simulink model "pattern3x3_training_2023clock"  (R2024a)
settings: Solver=FixedStepAuto  StartTime=0.0  StopTime=2  FixedStep=0.000005  RelTol=1e-3
model workspace (MAT data in the model file):
  part1_v1 = 1
values from neighbouring files (symbols this model uses):
  full_pattern = load('Pattern4_250.CSV')    [model_setup4.m]
  max_weight2 = 255    [model_setup4.m]
  min_weight2 = 150    [model_setup4.m]
  Th_minus_count2 = 10    [model_setup4.m]    (also in model_setup_test.m = 5)
  Th_plus_count2 = 20    [model_setup4.m]    (also in model_setup_test.m)
libraries: simulink x1
(part 5 of 9)

== system pattern3x3_training_2023clock/Neuron4/Clock4 ==
  clock : Inport
  "Reset " : Inport  Port=2
  Memory2 : Memory
  NOT1 : Logic  Operator=NOT  IconShape=distinctive  AllPortsSameDT=off  OutDataTypeStr=boolean
  Product1 : Product
  Scope4 : Scope  NumInputPorts=4
  Triggered Subsystem1 : Subsystem  TreatAsAtomicUnit=on
  T : Outport  VectorParamsAs1DForOutWhenUnconnected=off
  wires:
  Memory2/1 -> Triggered Subsystem1/1(In1)
  Product1/1 -> Scope4/4, T/1, Memory2/1
  "Reset "/1 -> Scope4/2, NOT1/1
  Triggered Subsystem1/1(Out1) -> Scope4/3, Product1/1
  NOT1/1 -> Product1/2
  clock/1 -> Scope4/1, Triggered Subsystem1/Trigger

== system pattern3x3_training_2023clock/Neuron4/Subsystem2 ==
  note: 기존 membrane potential + input potential
  Input potential : Inport
  before_Potential : Inport  Port=2
  Trigger : TriggerPort  VariantControl=(inherit)  PortDimensions=1
  Sum : Sum  Inputs=|++
  membrane_state : Outport
  wires:
  Input potential/1 -> Sum/1
  Sum/1 -> membrane_state/1
  before_Potential/1 -> Sum/2

== system pattern3x3_training_2023clock/Neuron4/Subsystem3 ==
  spike : Inport  OutDataTypeStr=double
  initial_threshold : Inport  Port=2
  neuron_num : Inport  Port=3
  clock : Inport  Port=4
  Add1 : Sum
  Constant2 : Constant  Value=0
  Delay : Delay  DelayLength=1  SampleTime=0.00001
  Delay1 : Delay  DelayLength=1  SampleTime=0.00001
  From Workspace3 : FromWorkspace  VariableName=Th_plus
  From Workspace4 : FromWorkspace  VariableName=Th_minus
  From Workspace5 : FromWorkspace  VariableName=Th_mean_count
  From Workspace6 : FromWorkspace  VariableName=min_th
  From Workspace7 : FromWorkspace  VariableName=max_th
  MATLAB Function : MATLAB Function  TreatAsAtomicUnit=on
  MATLAB Function2 : MATLAB Function  TreatAsAtomicUnit=on
  Memory2 : Memory
  NOT : Logic  Operator=NOT  IconShape=distinctive  AllPortsSameDT=off  OutDataTypeStr=boolean
  Product : Product
  Product1 : Product
  Scope1 : Scope  NumInputPorts=3
  Scope2 : Scope  NumInputPorts=3
  Scope3 : Scope  NumInputPorts=3
  Scope4 : Scope  NumInputPorts=4
  Sum : Sum  Inputs=++|
  Sum1 : Sum  Inputs=|++
  Switch3 : Switch  Criteria=u2 > Threshold  SaturateOnIntegerOverflow=off  InputSameDT=off
  Switch4 : Switch  Threshold=Th_plus_count2  SaturateOnIntegerOverflow=off  InputSameDT=off
  Switch5 : Switch  Threshold=Th_minus_count2  SaturateOnIntegerOverflow=off  InputSameDT=off
  clock_0.02 : Subsystem
  spike_generator2 : Subsystem
  Threshold : Outport
  wires:
  MATLAB Function2/1(y) -> Scope3/1, Sum/2
  Sum/1 -> MATLAB Function/1(u)  "Threshold"
  From Workspace7/1 -> MATLAB Function/3(max)
  Delay1/1 -> Scope3/3, MATLAB Function2/3(before_threshold)
  neuron_num/1 -> MATLAB Function2/2(neuron_num)
  MATLAB Function/1(y) -> Delay1/1, Scope3/2, Threshold/1
  initial_threshold/1 -> MATLAB Function2/1(init_th)
  From Workspace6/1 -> MATLAB Function/2(min)
  clock_0.02/1(clock) -> Switch3/2, Scope4/1, Product1/1, NOT/1
  Product1/1 -> Scope2/2, Scope4/2, spike_generator2/1(del_th)
  spike/1 -> Scope2/1, Sum1/1
  Delay/1 -> Sum1/2
  Product/1 -> Delay/1, Scope2/3
  Switch4/1 -> Add1/1, Scope1/1
  Switch5/1 -> Scope1/3, Add1/2
  Sum1/1 -> Product1/2, Product/2
  Constant2/1 -> Switch5/1, Switch4/3
  From Workspace4/1 -> Switch5/3
  Switch3/1 -> Scope4/4, Switch5/2, Switch4/2
  From Workspace3/1 -> Switch4/1
  NOT/1 -> Product/1
  spike_generator2/1(del_th_spike) -> Switch3/1, Scope4/3
  From Workspace5/1 -> Switch3/3
  Memory2/1 -> Scope1/2, Sum/1
  Add1/1 -> Memory2/1
  clock/1 -> clock_0.02/1(In1)

== system pattern3x3_training_2023clock/Neuron4/spike_generator1 ==
  1 : Inport
  AND : Logic  IconShape=distinctive  AllPortsSameDT=off  OutDataTypeStr=boolean
  Cast To Double : DataTypeConversion  OutDataTypeStr=double  SaturateOnIntegerOverflow=off  RndMeth=Floor
  Delay1 : Delay
  NOT : Logic  Operator=NOT  IconShape=distinctive  AllPortsSameDT=off  OutDataTypeStr=boolean
  Scope3 : Scope  NumInputPorts=5
  spike : Outport
  wires:
  NOT/1 -> Scope3/2, Delay1/1
  Delay1/1 -> Scope3/3, AND/2
  AND/1 -> Scope3/4, Cast To Double/1
  1/1 -> AND/1, Scope3/1, NOT/1
  Cast To Double/1 -> Scope3/5, spike/1

== system pattern3x3_training_2023clock/Neuron5/Clock4 ==
  clock : Inport
  "Reset " : Inport  Port=2
  Memory2 : Memory
  NOT1 : Logic  Operator=NOT  IconShape=distinctive  AllPortsSameDT=off  OutDataTypeStr=boolean
  Product1 : Product
  Scope4 : Scope  NumInputPorts=4
  Triggered Subsystem1 : Subsystem  TreatAsAtomicUnit=on
  T : Outport  VectorParamsAs1DForOutWhenUnconnected=off
  wires:
  Memory2/1 -> Triggered Subsystem1/1(In1)
  Product1/1 -> Scope4/4, T/1, Memory2/1
  "Reset "/1 -> Scope4/2, NOT1/1
  Triggered Subsystem1/1(Out1) -> Scope4/3, Product1/1
  NOT1/1 -> Product1/2
  clock/1 -> Scope4/1, Triggered Subsystem1/Trigger

== system pattern3x3_training_2023clock/Neuron5/Subsystem2 ==
  note: 기존 membrane potential + input potential
  Input potential : Inport
  before_Potential : Inport  Port=2
  Trigger : TriggerPort  VariantControl=(inherit)  PortDimensions=1
  Sum : Sum  Inputs=|++
  membrane_state : Outport
  wires:
  Input potential/1 -> Sum/1
  Sum/1 -> membrane_state/1
  before_Potential/1 -> Sum/2

== system pattern3x3_training_2023clock/Neuron5/Subsystem3 ==
  spike : Inport  OutDataTypeStr=double
  initial_threshold : Inport  Port=2
  neuron_num : Inport  Port=3
  clock : Inport  Port=4
  Add1 : Sum
  Constant2 : Constant  Value=0
  Delay : Delay  DelayLength=1  SampleTime=0.00001
  Delay1 : Delay  DelayLength=1  SampleTime=0.00001
  From Workspace3 : FromWorkspace  VariableName=Th_plus
  From Workspace4 : FromWorkspace  VariableName=Th_minus
  From Workspace5 : FromWorkspace  VariableName=Th_mean_count
  From Workspace6 : FromWorkspace  VariableName=min_th
  From Workspace7 : FromWorkspace  VariableName=max_th
  MATLAB Function : MATLAB Function  TreatAsAtomicUnit=on
  MATLAB Function2 : MATLAB Function  TreatAsAtomicUnit=on
  Memory2 : Memory
  NOT : Logic  Operator=NOT  IconShape=distinctive  AllPortsSameDT=off  OutDataTypeStr=boolean
  Product : Product
  Product1 : Product
  Scope1 : Scope  NumInputPorts=3
  Scope2 : Scope  NumInputPorts=3
  Scope3 : Scope  NumInputPorts=3
  Scope4 : Scope  NumInputPorts=4
  Sum : Sum  Inputs=++|
  Sum1 : Sum  Inputs=|++
  Switch3 : Switch  Criteria=u2 > Threshold  SaturateOnIntegerOverflow=off  InputSameDT=off
  Switch4 : Switch  Threshold=Th_plus_count2  SaturateOnIntegerOverflow=off  InputSameDT=off
  Switch5 : Switch  Threshold=Th_minus_count2  SaturateOnIntegerOverflow=off  InputSameDT=off
  clock_0.02 : Subsystem
  spike_generator2 : Subsystem
  Threshold : Outport
  wires:
  MATLAB Function2/1(y) -> Scope3/1, Sum/2
  Sum/1 -> MATLAB Function/1(u)  "Threshold"
  From Workspace7/1 -> MATLAB Function/3(max)
  Delay1/1 -> Scope3/3, MATLAB Function2/3(before_threshold)
  neuron_num/1 -> MATLAB Function2/2(neuron_num)
  MATLAB Function/1(y) -> Delay1/1, Scope3/2, Threshold/1
  initial_threshold/1 -> MATLAB Function2/1(init_th)
  From Workspace6/1 -> MATLAB Function/2(min)
  clock_0.02/1(clock) -> Switch3/2, Scope4/1, Product1/1, NOT/1
  Product1/1 -> Scope2/2, Scope4/2, spike_generator2/1(del_th)
  spike/1 -> Scope2/1, Sum1/1
  Delay/1 -> Sum1/2
  Product/1 -> Delay/1, Scope2/3
  Switch4/1 -> Add1/1, Scope1/1
  Switch5/1 -> Scope1/3, Add1/2
  Sum1/1 -> Product1/2, Product/2
  Constant2/1 -> Switch5/1, Switch4/3
  From Workspace4/1 -> Switch5/3
  Switch3/1 -> Scope4/4, Switch5/2, Switch4/2
  From Workspace3/1 -> Switch4/1
  NOT/1 -> Product/1
  spike_generator2/1(del_th_spike) -> Switch3/1, Scope4/3
  From Workspace5/1 -> Switch3/3
  Memory2/1 -> Scope1/2, Sum/1
  Add1/1 -> Memory2/1
  clock/1 -> clock_0.02/1(In1)

== system pattern3x3_training_2023clock/Neuron5/spike_generator1 ==
  1 : Inport
  AND : Logic  IconShape=distinctive  AllPortsSameDT=off  OutDataTypeStr=boolean
  Cast To Double : DataTypeConversion  OutDataTypeStr=double  SaturateOnIntegerOverflow=off  RndMeth=Floor
  Delay1 : Delay
  NOT : Logic  Operator=NOT  IconShape=distinctive  AllPortsSameDT=off  OutDataTypeStr=boolean
  Scope3 : Scope  NumInputPorts=5
  spike : Outport
  wires:
  NOT/1 -> Scope3/2, Delay1/1
  Delay1/1 -> Scope3/3, AND/2
  AND/1 -> Scope3/4, Cast To Double/1
  1/1 -> AND/1, Scope3/1, NOT/1
  Cast To Double/1 -> Scope3/5, spike/1

== system pattern3x3_training_2023clock/Neuron6/Clock4 ==
  clock : Inport
  "Reset " : Inport  Port=2
  Memory2 : Memory
  NOT1 : Logic  Operator=NOT  IconShape=distinctive  AllPortsSameDT=off  OutDataTypeStr=boolean
  Product1 : Product
  Scope4 : Scope  NumInputPorts=4
  Triggered Subsystem1 : Subsystem  TreatAsAtomicUnit=on
  T : Outport  VectorParamsAs1DForOutWhenUnconnected=off
  wires:
  Memory2/1 -> Triggered Subsystem1/1(In1)
  Product1/1 -> Scope4/4, T/1, Memory2/1
  "Reset "/1 -> Scope4/2, NOT1/1
  Triggered Subsystem1/1(Out1) -> Scope4/3, Product1/1
  NOT1/1 -> Product1/2
  clock/1 -> Scope4/1, Triggered Subsystem1/Trigger

== system pattern3x3_training_2023clock/Neuron6/Subsystem2 ==
  note: 기존 membrane potential + input potential
  Input potential : Inport
  before_Potential : Inport  Port=2
  Trigger : TriggerPort  VariantControl=(inherit)  PortDimensions=1
  Sum : Sum  Inputs=|++
  membrane_state : Outport
  wires:
  Input potential/1 -> Sum/1
  Sum/1 -> membrane_state/1
  before_Potential/1 -> Sum/2

== system pattern3x3_training_2023clock/Neuron6/Subsystem3 ==
  spike : Inport  OutDataTypeStr=double
  initial_threshold : Inport  Port=2
  neuron_num : Inport  Port=3
  clock : Inport  Port=4
  Add1 : Sum
  Constant2 : Constant  Value=0
  Delay : Delay  DelayLength=1  SampleTime=0.00001
  Delay1 : Delay  DelayLength=1  SampleTime=0.00001
  From Workspace3 : FromWorkspace  VariableName=Th_plus
  From Workspace4 : FromWorkspace  VariableName=Th_minus
  From Workspace5 : FromWorkspace  VariableName=Th_mean_count
  From Workspace6 : FromWorkspace  VariableName=min_th
  From Workspace7 : FromWorkspace  VariableName=max_th
  MATLAB Function : MATLAB Function  TreatAsAtomicUnit=on
  MATLAB Function2 : MATLAB Function  TreatAsAtomicUnit=on
  Memory2 : Memory
  NOT : Logic  Operator=NOT  IconShape=distinctive  AllPortsSameDT=off  OutDataTypeStr=boolean
  Product : Product
  Product1 : Product
  Scope1 : Scope  NumInputPorts=3
  Scope2 : Scope  NumInputPorts=3
  Scope3 : Scope  NumInputPorts=3
  Scope4 : Scope  NumInputPorts=4
  Sum : Sum  Inputs=++|
  Sum1 : Sum  Inputs=|++
  Switch3 : Switch  Criteria=u2 > Threshold  SaturateOnIntegerOverflow=off  InputSameDT=off
  Switch4 : Switch  Threshold=Th_plus_count2  SaturateOnIntegerOverflow=off  InputSameDT=off
  Switch5 : Switch  Threshold=Th_minus_count2  SaturateOnIntegerOverflow=off  InputSameDT=off
  clock_0.02 : Subsystem
  spike_generator2 : Subsystem
  Threshold : Outport
  wires:
  MATLAB Function2/1(y) -> Scope3/1, Sum/2
  Sum/1 -> MATLAB Function/1(u)  "Threshold"
  From Workspace7/1 -> MATLAB Function/3(max)
  Delay1/1 -> Scope3/3, MATLAB Function2/3(before_threshold)
  neuron_num/1 -> MATLAB Function2/2(neuron_num)
  MATLAB Function/1(y) -> Delay1/1, Scope3/2, Threshold/1
  initial_threshold/1 -> MATLAB Function2/1(init_th)
  From Workspace6/1 -> MATLAB Function/2(min)
  clock_0.02/1(clock) -> Switch3/2, Scope4/1, Product1/1, NOT/1
  Product1/1 -> Scope2/2, Scope4/2, spike_generator2/1(del_th)
  spike/1 -> Scope2/1, Sum1/1
  Delay/1 -> Sum1/2
  Product/1 -> Delay/1, Scope2/3
  Switch4/1 -> Add1/1, Scope1/1
  Switch5/1 -> Scope1/3, Add1/2
  Sum1/1 -> Product1/2, Product/2
  Constant2/1 -> Switch5/1, Switch4/3
  From Workspace4/1 -> Switch5/3
  Switch3/1 -> Scope4/4, Switch5/2, Switch4/2
  From Workspace3/1 -> Switch4/1
  NOT/1 -> Product/1
  spike_generator2/1(del_th_spike) -> Switch3/1, Scope4/3
  From Workspace5/1 -> Switch3/3
  Memory2/1 -> Scope1/2, Sum/1
  Add1/1 -> Memory2/1
  clock/1 -> clock_0.02/1(In1)

== system pattern3x3_training_2023clock/Neuron6/spike_generator1 ==
  1 : Inport
  AND : Logic  IconShape=distinctive  AllPortsSameDT=off  OutDataTypeStr=boolean
  Cast To Double : DataTypeConversion  OutDataTypeStr=double  SaturateOnIntegerOverflow=off  RndMeth=Floor
  Delay1 : Delay
  NOT : Logic  Operator=NOT  IconShape=distinctive  AllPortsSameDT=off  OutDataTypeStr=boolean
  Scope3 : Scope  NumInputPorts=5
  spike : Outport
  wires:
  NOT/1 -> Scope3/2, Delay1/1
  Delay1/1 -> Scope3/3, AND/2
  AND/1 -> Scope3/4, Cast To Double/1
  1/1 -> AND/1, Scope3/1, NOT/1
  Cast To Double/1 -> Scope3/5, spike/1

== system pattern3x3_training_2023clock/Neuron7/Clock4 ==
  clock : Inport
  "Reset " : Inport  Port=2
  Memory2 : Memory
  NOT1 : Logic  Operator=NOT  IconShape=distinctive  AllPortsSameDT=off  OutDataTypeStr=boolean
  Product1 : Product
  Scope4 : Scope  NumInputPorts=4
  Triggered Subsystem1 : Subsystem  TreatAsAtomicUnit=on
  T : Outport  VectorParamsAs1DForOutWhenUnconnected=off
  wires:
  Memory2/1 -> Triggered Subsystem1/1(In1)
  Product1/1 -> Scope4/4, T/1, Memory2/1
  "Reset "/1 -> Scope4/2, NOT1/1
  Triggered Subsystem1/1(Out1) -> Scope4/3, Product1/1
  NOT1/1 -> Product1/2
  clock/1 -> Scope4/1, Triggered Subsystem1/Trigger

== system pattern3x3_training_2023clock/Neuron7/Subsystem2 ==
  note: 기존 membrane potential + input potential
  Input potential : Inport
  before_Potential : Inport  Port=2
  Trigger : TriggerPort  VariantControl=(inherit)  PortDimensions=1
  Sum : Sum  Inputs=|++
  membrane_state : Outport
  wires:
  Input potential/1 -> Sum/1
  Sum/1 -> membrane_state/1
  before_Potential/1 -> Sum/2

== system pattern3x3_training_2023clock/Neuron7/Subsystem3 ==
  spike : Inport  OutDataTypeStr=double
  initial_threshold : Inport  Port=2
  neuron_num : Inport  Port=3
  clock : Inport  Port=4
  Add1 : Sum
  Constant2 : Constant  Value=0
  Delay : Delay  DelayLength=1  SampleTime=0.00001
  Delay1 : Delay  DelayLength=1  SampleTime=0.00001
  From Workspace3 : FromWorkspace  VariableName=Th_plus
  From Workspace4 : FromWorkspace  VariableName=Th_minus
  From Workspace5 : FromWorkspace  VariableName=Th_mean_count
  From Workspace6 : FromWorkspace  VariableName=min_th
  From Workspace7 : FromWorkspace  VariableName=max_th
  MATLAB Function : MATLAB Function  TreatAsAtomicUnit=on
  MATLAB Function2 : MATLAB Function  TreatAsAtomicUnit=on
  Memory2 : Memory
  NOT : Logic  Operator=NOT  IconShape=distinctive  AllPortsSameDT=off  OutDataTypeStr=boolean
  Product : Product
  Product1 : Product
  Scope1 : Scope  NumInputPorts=3
  Scope2 : Scope  NumInputPorts=3
  Scope3 : Scope  NumInputPorts=3
  Scope4 : Scope  NumInputPorts=4
  Sum : Sum  Inputs=++|
  Sum1 : Sum  Inputs=|++
  Switch3 : Switch  Criteria=u2 > Threshold  SaturateOnIntegerOverflow=off  InputSameDT=off
  Switch4 : Switch  Threshold=Th_plus_count2  SaturateOnIntegerOverflow=off  InputSameDT=off
  Switch5 : Switch  Threshold=Th_minus_count2  SaturateOnIntegerOverflow=off  InputSameDT=off
  clock_0.02 : Subsystem
  spike_generator2 : Subsystem
  Threshold : Outport
  wires:
  MATLAB Function2/1(y) -> Scope3/1, Sum/2
  Sum/1 -> MATLAB Function/1(u)  "Threshold"
  From Workspace7/1 -> MATLAB Function/3(max)
  Delay1/1 -> Scope3/3, MATLAB Function2/3(before_threshold)
  neuron_num/1 -> MATLAB Function2/2(neuron_num)
  MATLAB Function/1(y) -> Delay1/1, Scope3/2, Threshold/1
  initial_threshold/1 -> MATLAB Function2/1(init_th)
  From Workspace6/1 -> MATLAB Function/2(min)
  clock_0.02/1(clock) -> Switch3/2, Scope4/1, Product1/1, NOT/1
  Product1/1 -> Scope2/2, Scope4/2, spike_generator2/1(del_th)
  spike/1 -> Scope2/1, Sum1/1
  Delay/1 -> Sum1/2
  Product/1 -> Delay/1, Scope2/3
  Switch4/1 -> Add1/1, Scope1/1
  Switch5/1 -> Scope1/3, Add1/2
  Sum1/1 -> Product1/2, Product/2
  Constant2/1 -> Switch5/1, Switch4/3
  From Workspace4/1 -> Switch5/3
  Switch3/1 -> Scope4/4, Switch5/2, Switch4/2
  From Workspace3/1 -> Switch4/1
  NOT/1 -> Product/1
  spike_generator2/1(del_th_spike) -> Switch3/1, Scope4/3
  From Workspace5/1 -> Switch3/3
  Memory2/1 -> Scope1/2, Sum/1
  Add1/1 -> Memory2/1
  clock/1 -> clock_0.02/1(In1)

== system pattern3x3_training_2023clock/Neuron7/spike_generator1 ==
  1 : Inport
  AND : Logic  IconShape=distinctive  AllPortsSameDT=off  OutDataTypeStr=boolean
  Cast To Double : DataTypeConversion  OutDataTypeStr=double  SaturateOnIntegerOverflow=off  RndMeth=Floor
  Delay1 : Delay
  NOT : Logic  Operator=NOT  IconShape=distinctive  AllPortsSameDT=off  OutDataTypeStr=boolean
  Scope3 : Scope  NumInputPorts=5
  spike : Outport
  wires:
  NOT/1 -> Scope3/2, Delay1/1
  Delay1/1 -> Scope3/3, AND/2
  AND/1 -> Scope3/4, Cast To Double/1
  1/1 -> AND/1, Scope3/1, NOT/1
  Cast To Double/1 -> Scope3/5, spike/1

== system pattern3x3_training_2023clock/Neuron8/Clock4 ==
  clock : Inport
  "Reset " : Inport  Port=2
  Memory2 : Memory
  NOT1 : Logic  Operator=NOT  IconShape=distinctive  AllPortsSameDT=off  OutDataTypeStr=boolean
  Product1 : Product
  Scope4 : Scope  NumInputPorts=4
  Triggered Subsystem1 : Subsystem  TreatAsAtomicUnit=on
  T : Outport  VectorParamsAs1DForOutWhenUnconnected=off
  wires:
  Memory2/1 -> Triggered Subsystem1/1(In1)
  Product1/1 -> Scope4/4, T/1, Memory2/1
  "Reset "/1 -> Scope4/2, NOT1/1
  Triggered Subsystem1/1(Out1) -> Scope4/3, Product1/1
  NOT1/1 -> Product1/2
  clock/1 -> Scope4/1, Triggered Subsystem1/Trigger

== system pattern3x3_training_2023clock/Neuron8/Subsystem2 ==
  note: 기존 membrane potential + input potential
  Input potential : Inport
  before_Potential : Inport  Port=2
  Trigger : TriggerPort  VariantControl=(inherit)  PortDimensions=1
  Sum : Sum  Inputs=|++
  membrane_state : Outport
  wires:
  Input potential/1 -> Sum/1
  Sum/1 -> membrane_state/1
  before_Potential/1 -> Sum/2

== system pattern3x3_training_2023clock/Neuron8/Subsystem3 ==
  spike : Inport  OutDataTypeStr=double
  initial_threshold : Inport  Port=2
  neuron_num : Inport  Port=3
  clock : Inport  Port=4
  Add1 : Sum
  Constant2 : Constant  Value=0
  Delay : Delay  DelayLength=1  SampleTime=0.00001
  Delay1 : Delay  DelayLength=1  SampleTime=0.00001
  From Workspace3 : FromWorkspace  VariableName=Th_plus
  From Workspace4 : FromWorkspace  VariableName=Th_minus
  From Workspace5 : FromWorkspace  VariableName=Th_mean_count
  From Workspace6 : FromWorkspace  VariableName=min_th
  From Workspace7 : FromWorkspace  VariableName=max_th
  MATLAB Function : MATLAB Function  TreatAsAtomicUnit=on
  MATLAB Function2 : MATLAB Function  TreatAsAtomicUnit=on
  Memory2 : Memory
  NOT : Logic  Operator=NOT  IconShape=distinctive  AllPortsSameDT=off  OutDataTypeStr=boolean
  Product : Product
  Product1 : Product
  Scope1 : Scope  NumInputPorts=3
  Scope2 : Scope  NumInputPorts=3
  Scope3 : Scope  NumInputPorts=3
  Scope4 : Scope  NumInputPorts=4
  Sum : Sum  Inputs=++|
  Sum1 : Sum  Inputs=|++
  Switch3 : Switch  Criteria=u2 > Threshold  SaturateOnIntegerOverflow=off  InputSameDT=off
  Switch4 : Switch  Threshold=Th_plus_count2  SaturateOnIntegerOverflow=off  InputSameDT=off
  Switch5 : Switch  Threshold=Th_minus_count2  SaturateOnIntegerOverflow=off  InputSameDT=off
  clock_0.02 : Subsystem
  spike_generator2 : Subsystem
  Threshold : Outport
  wires:
  MATLAB Function2/1(y) -> Scope3/1, Sum/2
  Sum/1 -> MATLAB Function/1(u)  "Threshold"
  From Workspace7/1 -> MATLAB Function/3(max)
  Delay1/1 -> Scope3/3, MATLAB Function2/3(before_threshold)
  neuron_num/1 -> MATLAB Function2/2(neuron_num)
  MATLAB Function/1(y) -> Delay1/1, Scope3/2, Threshold/1
  initial_threshold/1 -> MATLAB Function2/1(init_th)
  From Workspace6/1 -> MATLAB Function/2(min)
  clock_0.02/1(clock) -> Switch3/2, Scope4/1, Product1/1, NOT/1
  Product1/1 -> Scope2/2, Scope4/2, spike_generator2/1(del_th)
  spike/1 -> Scope2/1, Sum1/1
  Delay/1 -> Sum1/2
  Product/1 -> Delay/1, Scope2/3
  Switch4/1 -> Add1/1, Scope1/1
  Switch5/1 -> Scope1/3, Add1/2
  Sum1/1 -> Product1/2, Product/2
  Constant2/1 -> Switch5/1, Switch4/3
  From Workspace4/1 -> Switch5/3
  Switch3/1 -> Scope4/4, Switch5/2, Switch4/2
  From Workspace3/1 -> Switch4/1
  NOT/1 -> Product/1
  spike_generator2/1(del_th_spike) -> Switch3/1, Scope4/3
  From Workspace5/1 -> Switch3/3
  Memory2/1 -> Scope1/2, Sum/1
  Add1/1 -> Memory2/1
  clock/1 -> clock_0.02/1(In1)

== system pattern3x3_training_2023clock/Neuron8/spike_generator1 ==
  1 : Inport
  AND : Logic  IconShape=distinctive  AllPortsSameDT=off  OutDataTypeStr=boolean
  Cast To Double : DataTypeConversion  OutDataTypeStr=double  SaturateOnIntegerOverflow=off  RndMeth=Floor
  Delay1 : Delay
  NOT : Logic  Operator=NOT  IconShape=distinctive  AllPortsSameDT=off  OutDataTypeStr=boolean
  Scope3 : Scope  NumInputPorts=5
  spike : Outport
  wires:
  NOT/1 -> Scope3/2, Delay1/1
  Delay1/1 -> Scope3/3, AND/2
  AND/1 -> Scope3/4, Cast To Double/1
  1/1 -> AND/1, Scope3/1, NOT/1
  Cast To Double/1 -> Scope3/5, spike/1

== system pattern3x3_training_2023clock/Neuron9/Clock4 ==
  clock : Inport
  "Reset " : Inport  Port=2
  Memory2 : Memory
  NOT1 : Logic  Operator=NOT  IconShape=distinctive  AllPortsSameDT=off  OutDataTypeStr=boolean
  Product1 : Product
  Scope4 : Scope  NumInputPorts=4
  Triggered Subsystem1 : Subsystem  TreatAsAtomicUnit=on
  T : Outport  VectorParamsAs1DForOutWhenUnconnected=off
  wires:
  Memory2/1 -> Triggered Subsystem1/1(In1)
  Product1/1 -> Scope4/4, T/1, Memory2/1
  "Reset "/1 -> Scope4/2, NOT1/1
  Triggered Subsystem1/1(Out1) -> Scope4/3, Product1/1
  NOT1/1 -> Product1/2
  clock/1 -> Scope4/1, Triggered Subsystem1/Trigger

== system pattern3x3_training_2023clock/Neuron9/Subsystem2 ==
  note: 기존 membrane potential + input potential
  Input potential : Inport
  before_Potential : Inport  Port=2
  Trigger : TriggerPort  VariantControl=(inherit)  PortDimensions=1
  Sum : Sum  Inputs=|++
  membrane_state : Outport
  wires:
  Input potential/1 -> Sum/1
  Sum/1 -> membrane_state/1
  before_Potential/1 -> Sum/2

== system pattern3x3_training_2023clock/Neuron9/Subsystem3 ==
  spike : Inport  OutDataTypeStr=double
  initial_threshold : Inport  Port=2
  neuron_num : Inport  Port=3
  clock : Inport  Port=4
  Add1 : Sum
  Constant2 : Constant  Value=0
  Delay : Delay  DelayLength=1  SampleTime=0.00001
  Delay1 : Delay  DelayLength=1  SampleTime=0.00001
  From Workspace3 : FromWorkspace  VariableName=Th_plus
  From Workspace4 : FromWorkspace  VariableName=Th_minus
  From Workspace5 : FromWorkspace  VariableName=Th_mean_count
  From Workspace6 : FromWorkspace  VariableName=min_th
  From Workspace7 : FromWorkspace  VariableName=max_th
  MATLAB Function : MATLAB Function  TreatAsAtomicUnit=on
  MATLAB Function2 : MATLAB Function  TreatAsAtomicUnit=on
  Memory2 : Memory
  NOT : Logic  Operator=NOT  IconShape=distinctive  AllPortsSameDT=off  OutDataTypeStr=boolean
  Product : Product
  Product1 : Product
  Scope1 : Scope  NumInputPorts=3
  Scope2 : Scope  NumInputPorts=3
  Scope3 : Scope  NumInputPorts=3
  Scope4 : Scope  NumInputPorts=4
  Sum : Sum  Inputs=++|
  Sum1 : Sum  Inputs=|++
  Switch3 : Switch  Criteria=u2 > Threshold  SaturateOnIntegerOverflow=off  InputSameDT=off
  Switch4 : Switch  Threshold=Th_plus_count2  SaturateOnIntegerOverflow=off  InputSameDT=off
  Switch5 : Switch  Threshold=Th_minus_count2  SaturateOnIntegerOverflow=off  InputSameDT=off
  clock_0.02 : Subsystem
  spike_generator2 : Subsystem
  Threshold : Outport
  wires:
  MATLAB Function2/1(y) -> Scope3/1, Sum/2
  Sum/1 -> MATLAB Function/1(u)  "Threshold"
  From Workspace7/1 -> MATLAB Function/3(max)
  Delay1/1 -> Scope3/3, MATLAB Function2/3(before_threshold)
  neuron_num/1 -> MATLAB Function2/2(neuron_num)
  MATLAB Function/1(y) -> Delay1/1, Scope3/2, Threshold/1
  initial_threshold/1 -> MATLAB Function2/1(init_th)
  From Workspace6/1 -> MATLAB Function/2(min)
  clock_0.02/1(clock) -> Switch3/2, Scope4/1, Product1/1, NOT/1
  Product1/1 -> Scope2/2, Scope4/2, spike_generator2/1(del_th)
  spike/1 -> Scope2/1, Sum1/1
  Delay/1 -> Sum1/2
  Product/1 -> Delay/1, Scope2/3
  Switch4/1 -> Add1/1, Scope1/1
  Switch5/1 -> Scope1/3, Add1/2
  Sum1/1 -> Product1/2, Product/2
  Constant2/1 -> Switch5/1, Switch4/3
  From Workspace4/1 -> Switch5/3
  Switch3/1 -> Scope4/4, Switch5/2, Switch4/2
  From Workspace3/1 -> Switch4/1
  NOT/1 -> Product/1
  spike_generator2/1(del_th_spike) -> Switch3/1, Scope4/3
  From Workspace5/1 -> Switch3/3
  Memory2/1 -> Scope1/2, Sum/1
  Add1/1 -> Memory2/1
  clock/1 -> clock_0.02/1(In1)

== system pattern3x3_training_2023clock/Neuron9/spike_generator1 ==
  1 : Inport
  AND : Logic  IconShape=distinctive  AllPortsSameDT=off  OutDataTypeStr=boolean
  Cast To Double : DataTypeConversion  OutDataTypeStr=double  SaturateOnIntegerOverflow=off  RndMeth=Floor
  Delay1 : Delay
  NOT : Logic  Operator=NOT  IconShape=distinctive  AllPortsSameDT=off  OutDataTypeStr=boolean
  Scope3 : Scope  NumInputPorts=5
  spike : Outport
  wires:
  NOT/1 -> Scope3/2, Delay1/1
  Delay1/1 -> Scope3/3, AND/2
  AND/1 -> Scope3/4, Cast To Double/1
  1/1 -> AND/1, Scope3/1, NOT/1
  Cast To Double/1 -> Scope3/5, spike/1

== system pattern3x3_training_2023clock/Post_Neuron1/Clock1 ==
  clock : Inport
  "Reset " : Inport  Port=2
  Memory2 : Memory
  NOT1 : Logic  Operator=NOT  IconShape=distinctive  AllPortsSameDT=off  OutDataTypeStr=boolean
  Product1 : Product
  Triggered Subsystem1 : Subsystem  TreatAsAtomicUnit=on
  T : Outport  VectorParamsAs1DForOutWhenUnconnected=off
  wires:
  Memory2/1 -> Triggered Subsystem1/1(In1)
  Product1/1 -> T/1, Memory2/1
  "Reset "/1 -> NOT1/1
  Triggered Subsystem1/1(Out1) -> Product1/1
  NOT1/1 -> Product1/2
  clock/1 -> Triggered Subsystem1/Trigger

== system pattern3x3_training_2023clock/Post_Neuron1/Clock2 ==
  clock : Inport
  "Reset " : Inport  Port=2
  Memory2 : Memory
  NOT1 : Logic  Operator=NOT  IconShape=distinctive  AllPortsSameDT=off  OutDataTypeStr=boolean
  Product1 : Product
  Triggered Subsystem1 : Subsystem  TreatAsAtomicUnit=on
  T : Outport  VectorParamsAs1DForOutWhenUnconnected=off
  wires:
  Memory2/1 -> Triggered Subsystem1/1(In1)
  Product1/1 -> T/1, Memory2/1
  "Reset "/1 -> NOT1/1
  Triggered Subsystem1/1(Out1) -> Product1/1
  NOT1/1 -> Product1/2
  clock/1 -> Triggered Subsystem1/Trigger

== system pattern3x3_training_2023clock/Post_Neuron1/Subsystem1 ==
  In1 : Inport
  In2 : Inport  Port=2
  Trigger : TriggerPort  VariantControl=(inherit)  PortDimensions=1
  Sum : Sum  Inputs=|++
  membrane_state : Outport
  wires:
  In1/1 -> Sum/1
  Sum/1 -> membrane_state/1
  In2/1 -> Sum/2

== system pattern3x3_training_2023clock/Post_Neuron1/Subsystem3 ==
  spike : Inport  OutDataTypeStr=double
  initial_threshold : Inport  Port=2
  neuron_num : Inport  Port=3
  clock : Inport  Port=4
  Add1 : Sum
  Constant2 : Constant  Value=0
  Delay : Delay  DelayLength=1  SampleTime=0.00001
  Delay1 : Delay  DelayLength=1  SampleTime=0.00001
  From Workspace3 : FromWorkspace  VariableName=Th_plus
  From Workspace4 : FromWorkspace  VariableName=Th_minus
  From Workspace5 : FromWorkspace  VariableName=Th_mean_count
  From Workspace6 : FromWorkspace  VariableName=min_th
  From Workspace7 : FromWorkspace  VariableName=max_th
  MATLAB Function : MATLAB Function  TreatAsAtomicUnit=on
  MATLAB Function2 : MATLAB Function  TreatAsAtomicUnit=on
  Memory2 : Memory
  NOT : Logic  Operator=NOT  IconShape=distinctive  AllPortsSameDT=off  OutDataTypeStr=boolean
  Product : Product
  Product1 : Product
  Scope1 : Scope  NumInputPorts=3
  Scope2 : Scope  NumInputPorts=3
  Scope3 : Scope  NumInputPorts=3
  Scope4 : Scope  NumInputPorts=4
  Sum : Sum  Inputs=++|
  Sum1 : Sum  Inputs=|++
  Switch3 : Switch  Criteria=u2 > Threshold  SaturateOnIntegerOverflow=off  InputSameDT=off
  Switch4 : Switch  Threshold=Th_plus_count2  SaturateOnIntegerOverflow=off  InputSameDT=off
  Switch5 : Switch  Threshold=Th_minus_count2  SaturateOnIntegerOverflow=off  InputSameDT=off
  clock_0.02 : Subsystem
  spike_generator2 : Subsystem
  Threshold : Outport
  wires:
  MATLAB Function2/1(y) -> Scope3/1, Sum/2
  Sum/1 -> MATLAB Function/1(u)  "Threshold"
  From Workspace7/1 -> MATLAB Function/3(max)
  Delay1/1 -> Scope3/3, MATLAB Function2/3(before_threshold)
  neuron_num/1 -> MATLAB Function2/2(neuron_num)
  MATLAB Function/1(y) -> Delay1/1, Scope3/2, Threshold/1
  initial_threshold/1 -> MATLAB Function2/1(init_th)
  From Workspace6/1 -> MATLAB Function/2(min)
  clock_0.02/1(clock) -> Switch3/2, Scope4/1, Product1/1, NOT/1
  Product1/1 -> Scope2/2, Scope4/2, spike_generator2/1(del_th)
  spike/1 -> Scope2/1, Sum1/1
  Delay/1 -> Sum1/2
  Product/1 -> Delay/1, Scope2/3
  Switch4/1 -> Add1/1, Scope1/1
  Switch5/1 -> Scope1/3, Add1/2
  Sum1/1 -> Product1/2, Product/2
  Constant2/1 -> Switch5/1, Switch4/3
  From Workspace4/1 -> Switch5/3
  Switch3/1 -> Scope4/4, Switch5/2, Switch4/2
  From Workspace3/1 -> Switch4/1
  NOT/1 -> Product/1
  spike_generator2/1(del_th_spike) -> Switch3/1, Scope4/3
  From Workspace5/1 -> Switch3/3
  Memory2/1 -> Scope1/2, Sum/1
  Add1/1 -> Memory2/1
  clock/1 -> clock_0.02/1(In1)

== system pattern3x3_training_2023clock/Post_Neuron1/memory ==
  In1 : Inport
  Memory2 : Memory
  Memory4 : Memory
  OR : Logic  Operator=OR  IconShape=distinctive  AllPortsSameDT=off  OutDataTypeStr=boolean
  Out1 : Outport
  wires:
  Memory4/1 -> Memory2/1, OR/1
  Memory2/1 -> OR/2
  OR/1 -> Out1/1
  In1/1 -> Memory4/1

== system pattern3x3_training_2023clock/Post_Neuron1/spike_generator1 ==
  1 : Inport
  AND : Logic  IconShape=distinctive  AllPortsSameDT=off  OutDataTypeStr=boolean
  Cast To Double : DataTypeConversion  OutDataTypeStr=double  SaturateOnIntegerOverflow=off  RndMeth=Floor
  Delay1 : Delay
  NOT : Logic  Operator=NOT  IconShape=distinctive  AllPortsSameDT=off  OutDataTypeStr=boolean
  Scope3 : Scope  NumInputPorts=5
  spike : Outport
  wires:
  NOT/1 -> Scope3/2, Delay1/1
  Delay1/1 -> Scope3/3, AND/2
  AND/1 -> Scope3/4, Cast To Double/1
  1/1 -> AND/1, Scope3/1, NOT/1
  Cast To Double/1 -> Scope3/5, spike/1

== system pattern3x3_training_2023clock/Post_Neuron2/Clock1 ==
  clock : Inport
  "Reset " : Inport  Port=2
  Memory2 : Memory
  NOT1 : Logic  Operator=NOT  IconShape=distinctive  AllPortsSameDT=off  OutDataTypeStr=boolean
  Product1 : Product
  Triggered Subsystem1 : Subsystem  TreatAsAtomicUnit=on
  T : Outport  VectorParamsAs1DForOutWhenUnconnected=off
  wires:
  Memory2/1 -> Triggered Subsystem1/1(In1)
  Product1/1 -> T/1, Memory2/1
  "Reset "/1 -> NOT1/1
  Triggered Subsystem1/1(Out1) -> Product1/1
  NOT1/1 -> Product1/2
  clock/1 -> Triggered Subsystem1/Trigger

== system pattern3x3_training_2023clock/Post_Neuron2/Clock2 ==
  clock : Inport
  "Reset " : Inport  Port=2
  Memory2 : Memory
  NOT1 : Logic  Operator=NOT  IconShape=distinctive  AllPortsSameDT=off  OutDataTypeStr=boolean
  Product1 : Product
  Triggered Subsystem1 : Subsystem  TreatAsAtomicUnit=on
  T : Outport  VectorParamsAs1DForOutWhenUnconnected=off
  wires:
  Memory2/1 -> Triggered Subsystem1/1(In1)
  Product1/1 -> T/1, Memory2/1
  "Reset "/1 -> NOT1/1
  Triggered Subsystem1/1(Out1) -> Product1/1
  NOT1/1 -> Product1/2
  clock/1 -> Triggered Subsystem1/Trigger

== system pattern3x3_training_2023clock/Post_Neuron2/Subsystem1 ==
  In1 : Inport
  In2 : Inport  Port=2
  Trigger : TriggerPort  VariantControl=(inherit)  PortDimensions=1
  Sum : Sum  Inputs=|++
  membrane_state : Outport
  wires:
  In1/1 -> Sum/1
  Sum/1 -> membrane_state/1
  In2/1 -> Sum/2

== system pattern3x3_training_2023clock/Post_Neuron2/Subsystem3 ==
  spike : Inport  OutDataTypeStr=double
  initial_threshold : Inport  Port=2
  neuron_num : Inport  Port=3
  clock : Inport  Port=4
  Add1 : Sum
  Constant2 : Constant  Value=0
  Delay : Delay  DelayLength=1  SampleTime=0.00001
  Delay1 : Delay  DelayLength=1  SampleTime=0.00001
  From Workspace3 : FromWorkspace  VariableName=Th_plus
  From Workspace4 : FromWorkspace  VariableName=Th_minus
  From Workspace5 : FromWorkspace  VariableName=Th_mean_count
  From Workspace6 : FromWorkspace  VariableName=min_th
  From Workspace7 : FromWorkspace  VariableName=max_th
  MATLAB Function : MATLAB Function  TreatAsAtomicUnit=on
  MATLAB Function2 : MATLAB Function  TreatAsAtomicUnit=on
  Memory2 : Memory
  NOT : Logic  Operator=NOT  IconShape=distinctive  AllPortsSameDT=off  OutDataTypeStr=boolean
  Product : Product
  Product1 : Product
  Scope1 : Scope  NumInputPorts=3
  Scope2 : Scope  NumInputPorts=3
  Scope3 : Scope  NumInputPorts=3
  Scope4 : Scope  NumInputPorts=4
  Sum : Sum  Inputs=++|
  Sum1 : Sum  Inputs=|++
  Switch3 : Switch  Criteria=u2 > Threshold  SaturateOnIntegerOverflow=off  InputSameDT=off
  Switch4 : Switch  Threshold=Th_plus_count2  SaturateOnIntegerOverflow=off  InputSameDT=off
  Switch5 : Switch  Threshold=Th_minus_count2  SaturateOnIntegerOverflow=off  InputSameDT=off
  clock_0.02 : Subsystem
  spike_generator2 : Subsystem
  Threshold : Outport
  wires:
  MATLAB Function2/1(y) -> Scope3/1, Sum/2
  Sum/1 -> MATLAB Function/1(u)  "Threshold"
  From Workspace7/1 -> MATLAB Function/3(max)
  Delay1/1 -> Scope3/3, MATLAB Function2/3(before_threshold)
  neuron_num/1 -> MATLAB Function2/2(neuron_num)
  MATLAB Function/1(y) -> Delay1/1, Scope3/2, Threshold/1
  initial_threshold/1 -> MATLAB Function2/1(init_th)
  From Workspace6/1 -> MATLAB Function/2(min)
  clock_0.02/1(clock) -> Switch3/2, Scope4/1, Product1/1, NOT/1
  Product1/1 -> Scope2/2, Scope4/2, spike_generator2/1(del_th)
  spike/1 -> Scope2/1, Sum1/1
  Delay/1 -> Sum1/2
  Product/1 -> Delay/1, Scope2/3
  Switch4/1 -> Add1/1, Scope1/1
  Switch5/1 -> Scope1/3, Add1/2
  Sum1/1 -> Product1/2, Product/2
  Constant2/1 -> Switch5/1, Switch4/3
  From Workspace4/1 -> Switch5/3
  Switch3/1 -> Scope4/4, Switch5/2, Switch4/2
  From Workspace3/1 -> Switch4/1
  NOT/1 -> Product/1
  spike_generator2/1(del_th_spike) -> Switch3/1, Scope4/3
  From Workspace5/1 -> Switch3/3
  Memory2/1 -> Scope1/2, Sum/1
  Add1/1 -> Memory2/1
  clock/1 -> clock_0.02/1(In1)

== system pattern3x3_training_2023clock/Post_Neuron2/memory ==
  In1 : Inport
  Memory2 : Memory
  Memory4 : Memory
  OR : Logic  Operator=OR  IconShape=distinctive  AllPortsSameDT=off  OutDataTypeStr=boolean
  Out1 : Outport
  wires:
  Memory4/1 -> Memory2/1, OR/1
  Memory2/1 -> OR/2
  OR/1 -> Out1/1
  In1/1 -> Memory4/1

== system pattern3x3_training_2023clock/Post_Neuron2/spike_generator1 ==
  1 : Inport
  AND : Logic  IconShape=distinctive  AllPortsSameDT=off  OutDataTypeStr=boolean
  Cast To Double : DataTypeConversion  OutDataTypeStr=double  SaturateOnIntegerOverflow=off  RndMeth=Floor
  Delay1 : Delay
  NOT : Logic  Operator=NOT  IconShape=distinctive  AllPortsSameDT=off  OutDataTypeStr=boolean
  Scope3 : Scope  NumInputPorts=5
  spike : Outport
  wires:
  NOT/1 -> Scope3/2, Delay1/1
  Delay1/1 -> Scope3/3, AND/2
  AND/1 -> Scope3/4, Cast To Double/1
  1/1 -> AND/1, Scope3/1, NOT/1
  Cast To Double/1 -> Scope3/5, spike/1

== system pattern3x3_training_2023clock/Post_Neuron3/Clock1 ==
  clock : Inport
  "Reset " : Inport  Port=2
  Memory2 : Memory
  NOT1 : Logic  Operator=NOT  IconShape=distinctive  AllPortsSameDT=off  OutDataTypeStr=boolean
  Product1 : Product
  Triggered Subsystem1 : Subsystem  TreatAsAtomicUnit=on
  T : Outport  VectorParamsAs1DForOutWhenUnconnected=off
  wires:
  Memory2/1 -> Triggered Subsystem1/1(In1)
  Product1/1 -> T/1, Memory2/1
  "Reset "/1 -> NOT1/1
  Triggered Subsystem1/1(Out1) -> Product1/1
  NOT1/1 -> Product1/2
  clock/1 -> Triggered Subsystem1/Trigger

== system pattern3x3_training_2023clock/Post_Neuron3/Clock2 ==
  clock : Inport
  "Reset " : Inport  Port=2
  Memory2 : Memory
  NOT1 : Logic  Operator=NOT  IconShape=distinctive  AllPortsSameDT=off  OutDataTypeStr=boolean
  Product1 : Product
  Triggered Subsystem1 : Subsystem  TreatAsAtomicUnit=on
  T : Outport  VectorParamsAs1DForOutWhenUnconnected=off
  wires:
  Memory2/1 -> Triggered Subsystem1/1(In1)
  Product1/1 -> T/1, Memory2/1
  "Reset "/1 -> NOT1/1
  Triggered Subsystem1/1(Out1) -> Product1/1
  NOT1/1 -> Product1/2
  clock/1 -> Triggered Subsystem1/Trigger

== system pattern3x3_training_2023clock/Post_Neuron3/Subsystem1 ==
  In1 : Inport
  In2 : Inport  Port=2
  Trigger : TriggerPort  VariantControl=(inherit)  PortDimensions=1
  Sum : Sum  Inputs=|++
  membrane_state : Outport
  wires:
  In1/1 -> Sum/1
  Sum/1 -> membrane_state/1
  In2/1 -> Sum/2

== system pattern3x3_training_2023clock/Post_Neuron3/Subsystem3 ==
  spike : Inport  OutDataTypeStr=double
  initial_threshold : Inport  Port=2
  neuron_num : Inport  Port=3
  clock : Inport  Port=4
  Add1 : Sum
  Constant2 : Constant  Value=0
  Delay : Delay  DelayLength=1  SampleTime=0.00001
  Delay1 : Delay  DelayLength=1  SampleTime=0.00001
  From Workspace3 : FromWorkspace  VariableName=Th_plus
  From Workspace4 : FromWorkspace  VariableName=Th_minus
  From Workspace5 : FromWorkspace  VariableName=Th_mean_count
  From Workspace6 : FromWorkspace  VariableName=min_th
  From Workspace7 : FromWorkspace  VariableName=max_th
  MATLAB Function : MATLAB Function  TreatAsAtomicUnit=on
  MATLAB Function2 : MATLAB Function  TreatAsAtomicUnit=on
  Memory2 : Memory
  NOT : Logic  Operator=NOT  IconShape=distinctive  AllPortsSameDT=off  OutDataTypeStr=boolean
  Product : Product
  Product1 : Product
  Scope1 : Scope  NumInputPorts=3
  Scope2 : Scope  NumInputPorts=3
  Scope3 : Scope  NumInputPorts=3
  Scope4 : Scope  NumInputPorts=4
  Sum : Sum  Inputs=++|
  Sum1 : Sum  Inputs=|++
  Switch3 : Switch  Criteria=u2 > Threshold  SaturateOnIntegerOverflow=off  InputSameDT=off
  Switch4 : Switch  Threshold=Th_plus_count2  SaturateOnIntegerOverflow=off  InputSameDT=off
  Switch5 : Switch  Threshold=Th_minus_count2  SaturateOnIntegerOverflow=off  InputSameDT=off
  clock_0.02 : Subsystem
  spike_generator2 : Subsystem
  Threshold : Outport
  wires:
  MATLAB Function2/1(y) -> Scope3/1, Sum/2
  Sum/1 -> MATLAB Function/1(u)  "Threshold"
  From Workspace7/1 -> MATLAB Function/3(max)
  Delay1/1 -> Scope3/3, MATLAB Function2/3(before_threshold)
  neuron_num/1 -> MATLAB Function2/2(neuron_num)
  MATLAB Function/1(y) -> Delay1/1, Scope3/2, Threshold/1
  initial_threshold/1 -> MATLAB Function2/1(init_th)
  From Workspace6/1 -> MATLAB Function/2(min)
  clock_0.02/1(clock) -> Switch3/2, Scope4/1, Product1/1, NOT/1
  Product1/1 -> Scope2/2, Scope4/2, spike_generator2/1(del_th)
  spike/1 -> Scope2/1, Sum1/1
  Delay/1 -> Sum1/2
  Product/1 -> Delay/1, Scope2/3
  Switch4/1 -> Add1/1, Scope1/1
  Switch5/1 -> Scope1/3, Add1/2
  Sum1/1 -> Product1/2, Product/2
  Constant2/1 -> Switch5/1, Switch4/3
  From Workspace4/1 -> Switch5/3
  Switch3/1 -> Scope4/4, Switch5/2, Switch4/2
  From Workspace3/1 -> Switch4/1
  NOT/1 -> Product/1
  spike_generator2/1(del_th_spike) -> Switch3/1, Scope4/3
  From Workspace5/1 -> Switch3/3
  Memory2/1 -> Scope1/2, Sum/1
  Add1/1 -> Memory2/1
  clock/1 -> clock_0.02/1(In1)

== system pattern3x3_training_2023clock/Post_Neuron3/memory ==
  In1 : Inport
  Memory2 : Memory
  Memory4 : Memory
  OR : Logic  Operator=OR  IconShape=distinctive  AllPortsSameDT=off  OutDataTypeStr=boolean
  Out1 : Outport
  wires:
  Memory4/1 -> Memory2/1, OR/1
  Memory2/1 -> OR/2
  OR/1 -> Out1/1
  In1/1 -> Memory4/1

== system pattern3x3_training_2023clock/Post_Neuron3/spike_generator1 ==
  1 : Inport
  AND : Logic  IconShape=distinctive  AllPortsSameDT=off  OutDataTypeStr=boolean
  Cast To Double : DataTypeConversion  OutDataTypeStr=double  SaturateOnIntegerOverflow=off  RndMeth=Floor
  Delay1 : Delay
  NOT : Logic  Operator=NOT  IconShape=distinctive  AllPortsSameDT=off  OutDataTypeStr=boolean
  Scope3 : Scope  NumInputPorts=5
  spike : Outport
  wires:
  NOT/1 -> Scope3/2, Delay1/1
  Delay1/1 -> Scope3/3, AND/2
  AND/1 -> Scope3/4, Cast To Double/1
  1/1 -> AND/1, Scope3/1, NOT/1
  Cast To Double/1 -> Scope3/5, spike/1

== system pattern3x3_training_2023clock/Post_Neuron4/Clock1 ==
  clock : Inport
  "Reset " : Inport  Port=2
  Memory2 : Memory
  NOT1 : Logic  Operator=NOT  IconShape=distinctive  AllPortsSameDT=off  OutDataTypeStr=boolean
  Product1 : Product
  Triggered Subsystem1 : Subsystem  TreatAsAtomicUnit=on
  T : Outport  VectorParamsAs1DForOutWhenUnconnected=off
  wires:
  Memory2/1 -> Triggered Subsystem1/1(In1)
  Product1/1 -> T/1, Memory2/1
  "Reset "/1 -> NOT1/1
  Triggered Subsystem1/1(Out1) -> Product1/1
  NOT1/1 -> Product1/2
  clock/1 -> Triggered Subsystem1/Trigger

== system pattern3x3_training_2023clock/Post_Neuron4/Clock2 ==
  clock : Inport
  "Reset " : Inport  Port=2
  Memory2 : Memory
  NOT1 : Logic  Operator=NOT  IconShape=distinctive  AllPortsSameDT=off  OutDataTypeStr=boolean
  Product1 : Product
  Triggered Subsystem1 : Subsystem  TreatAsAtomicUnit=on
  T : Outport  VectorParamsAs1DForOutWhenUnconnected=off
  wires:
  Memory2/1 -> Triggered Subsystem1/1(In1)
  Product1/1 -> T/1, Memory2/1
  "Reset "/1 -> NOT1/1
  Triggered Subsystem1/1(Out1) -> Product1/1
  NOT1/1 -> Product1/2
  clock/1 -> Triggered Subsystem1/Trigger

== system pattern3x3_training_2023clock/Post_Neuron4/Subsystem1 ==
  In1 : Inport
  In2 : Inport  Port=2
  Trigger : TriggerPort  VariantControl=(inherit)  PortDimensions=1
  Sum : Sum  Inputs=|++
  membrane_state : Outport
  wires:
  In1/1 -> Sum/1
  Sum/1 -> membrane_state/1
  In2/1 -> Sum/2

== system pattern3x3_training_2023clock/Post_Neuron4/Subsystem3 ==
  spike : Inport  OutDataTypeStr=double
  initial_threshold : Inport  Port=2
  neuron_num : Inport  Port=3
  clock : Inport  Port=4
  Add1 : Sum
  Constant2 : Constant  Value=0
  Delay : Delay  DelayLength=1  SampleTime=0.00001
  Delay1 : Delay  DelayLength=1  SampleTime=0.00001
  From Workspace3 : FromWorkspace  VariableName=Th_plus
  From Workspace4 : FromWorkspace  VariableName=Th_minus
  From Workspace5 : FromWorkspace  VariableName=Th_mean_count
  From Workspace6 : FromWorkspace  VariableName=min_th
  From Workspace7 : FromWorkspace  VariableName=max_th
  MATLAB Function : MATLAB Function  TreatAsAtomicUnit=on
  MATLAB Function2 : MATLAB Function  TreatAsAtomicUnit=on
  Memory2 : Memory
  NOT : Logic  Operator=NOT  IconShape=distinctive  AllPortsSameDT=off  OutDataTypeStr=boolean
  Product : Product
  Product1 : Product
  Scope1 : Scope  NumInputPorts=3
  Scope2 : Scope  NumInputPorts=3
  Scope3 : Scope  NumInputPorts=3
  Scope4 : Scope  NumInputPorts=4
  Sum : Sum  Inputs=++|
  Sum1 : Sum  Inputs=|++
  Switch3 : Switch  Criteria=u2 > Threshold  SaturateOnIntegerOverflow=off  InputSameDT=off
  Switch4 : Switch  Threshold=Th_plus_count2  SaturateOnIntegerOverflow=off  InputSameDT=off
  Switch5 : Switch  Threshold=Th_minus_count2  SaturateOnIntegerOverflow=off  InputSameDT=off
  clock_0.02 : Subsystem
  spike_generator2 : Subsystem
  Threshold : Outport
  wires:
  MATLAB Function2/1(y) -> Scope3/1, Sum/2
  Sum/1 -> MATLAB Function/1(u)  "Threshold"
  From Workspace7/1 -> MATLAB Function/3(max)
  Delay1/1 -> Scope3/3, MATLAB Function2/3(before_threshold)
  neuron_num/1 -> MATLAB Function2/2(neuron_num)
  MATLAB Function/1(y) -> Delay1/1, Scope3/2, Threshold/1
  initial_threshold/1 -> MATLAB Function2/1(init_th)
  From Workspace6/1 -> MATLAB Function/2(min)
  clock_0.02/1(clock) -> Switch3/2, Scope4/1, Product1/1, NOT/1
  Product1/1 -> Scope2/2, Scope4/2, spike_generator2/1(del_th)
  spike/1 -> Scope2/1, Sum1/1
  Delay/1 -> Sum1/2
  Product/1 -> Delay/1, Scope2/3
  Switch4/1 -> Add1/1, Scope1/1
  Switch5/1 -> Scope1/3, Add1/2
  Sum1/1 -> Product1/2, Product/2
  Constant2/1 -> Switch5/1, Switch4/3
  From Workspace4/1 -> Switch5/3
  Switch3/1 -> Scope4/4, Switch5/2, Switch4/2
  From Workspace3/1 -> Switch4/1
  NOT/1 -> Product/1
  spike_generator2/1(del_th_spike) -> Switch3/1, Scope4/3
  From Workspace5/1 -> Switch3/3
  Memory2/1 -> Scope1/2, Sum/1
  Add1/1 -> Memory2/1
  clock/1 -> clock_0.02/1(In1)

== system pattern3x3_training_2023clock/Post_Neuron4/memory ==
  In1 : Inport
  Memory2 : Memory
  Memory4 : Memory
  OR : Logic  Operator=OR  IconShape=distinctive  AllPortsSameDT=off  OutDataTypeStr=boolean
  Out1 : Outport
  wires:
  Memory4/1 -> Memory2/1, OR/1
  Memory2/1 -> OR/2
  OR/1 -> Out1/1
  In1/1 -> Memory4/1

== system pattern3x3_training_2023clock/Post_Neuron4/spike_generator1 ==
  1 : Inport
  AND : Logic  IconShape=distinctive  AllPortsSameDT=off  OutDataTypeStr=boolean
  Cast To Double : DataTypeConversion  OutDataTypeStr=double  SaturateOnIntegerOverflow=off  RndMeth=Floor
  Delay1 : Delay
  NOT : Logic  Operator=NOT  IconShape=distinctive  AllPortsSameDT=off  OutDataTypeStr=boolean
  Scope3 : Scope  NumInputPorts=5
  spike : Outport
  wires:
  NOT/1 -> Scope3/2, Delay1/1
  Delay1/1 -> Scope3/3, AND/2
  AND/1 -> Scope3/4, Cast To Double/1
  1/1 -> AND/1, Scope3/1, NOT/1
  Cast To Double/1 -> Scope3/5, spike/1

== system pattern3x3_training_2023clock/Synapse1/Clock1 ==
  clock : Inport
  "Reset " : Inport  Port=2
  Memory2 : Memory
  NOT1 : Logic  Operator=NOT  IconShape=distinctive  AllPortsSameDT=off  OutDataTypeStr=boolean
  Product1 : Product
  Triggered Subsystem1 : Subsystem  TreatAsAtomicUnit=on
  T : Outport  VectorParamsAs1DForOutWhenUnconnected=off
  wires:
  Memory2/1 -> Triggered Subsystem1/1(In1)
  Product1/1 -> T/1, Memory2/1
  "Reset "/1 -> NOT1/1
  Triggered Subsystem1/1(Out1) -> Product1/1
  NOT1/1 -> Product1/2
  clock/1 -> Triggered Subsystem1/Trigger

== system pattern3x3_training_2023clock/Synapse1/Clock2 ==
  clock : Inport
  "Reset " : Inport  Port=2
  Memory2 : Memory
  NOT1 : Logic  Operator=NOT  IconShape=distinctive  AllPortsSameDT=off  OutDataTypeStr=boolean
  Product1 : Product
  Triggered Subsystem1 : Subsystem  TreatAsAtomicUnit=on
  T : Outport  VectorParamsAs1DForOutWhenUnconnected=off
  wires:
  Memory2/1 -> Triggered Subsystem1/1(In1)
  Product1/1 -> T/1, Memory2/1
  "Reset "/1 -> NOT1/1
  Triggered Subsystem1/1(Out1) -> Product1/1
  NOT1/1 -> Product1/2
  clock/1 -> Triggered Subsystem1/Trigger

== system pattern3x3_training_2023clock/Synapse1/Clock3 ==
  clock : Inport
  "Reset " : Inport  Port=2
  Memory2 : Memory
  NOT1 : Logic  Operator=NOT  IconShape=distinctive  AllPortsSameDT=off  OutDataTypeStr=boolean
  Product1 : Product
  Triggered Subsystem1 : Subsystem  TreatAsAtomicUnit=on
  T : Outport  VectorParamsAs1DForOutWhenUnconnected=off
  wires:
  Memory2/1 -> Triggered Subsystem1/1(In1)
  Product1/1 -> T/1, Memory2/1
  "Reset "/1 -> NOT1/1
  Triggered Subsystem1/1(Out1) -> Product1/1
  NOT1/1 -> Product1/2
  clock/1 -> Triggered Subsystem1/Trigger

== system pattern3x3_training_2023clock/Synapse1/Subsystem ==
  delta_weight : Inport
  before_weight : Inport  Port=2
  Trigger : TriggerPort  VariantControl=(inherit)  PortDimensions=1
  Sum : Sum  Inputs=|++
  weight : Outport
  wires:
  delta_weight/1 -> Sum/1
  Sum/1 -> weight/1
  before_weight/1 -> Sum/2

== system pattern3x3_training_2023clock/Synapse10/Clock1 ==
  clock : Inport
  "Reset " : Inport  Port=2
  Memory2 : Memory
  NOT1 : Logic  Operator=NOT  IconShape=distinctive  AllPortsSameDT=off  OutDataTypeStr=boolean
  Product1 : Product
  Triggered Subsystem1 : Subsystem  TreatAsAtomicUnit=on
  T : Outport  VectorParamsAs1DForOutWhenUnconnected=off
  wires:
  Memory2/1 -> Triggered Subsystem1/1(In1)
  Product1/1 -> T/1, Memory2/1
  "Reset "/1 -> NOT1/1
  Triggered Subsystem1/1(Out1) -> Product1/1
  NOT1/1 -> Product1/2
  clock/1 -> Triggered Subsystem1/Trigger

== system pattern3x3_training_2023clock/Synapse10/Clock2 ==
  clock : Inport
  "Reset " : Inport  Port=2
  Memory2 : Memory
  NOT1 : Logic  Operator=NOT  IconShape=distinctive  AllPortsSameDT=off  OutDataTypeStr=boolean
  Product1 : Product
  Triggered Subsystem1 : Subsystem  TreatAsAtomicUnit=on
  T : Outport  VectorParamsAs1DForOutWhenUnconnected=off
  wires:
  Memory2/1 -> Triggered Subsystem1/1(In1)
  Product1/1 -> T/1, Memory2/1
  "Reset "/1 -> NOT1/1
  Triggered Subsystem1/1(Out1) -> Product1/1
  NOT1/1 -> Product1/2
  clock/1 -> Triggered Subsystem1/Trigger

== system pattern3x3_training_2023clock/Synapse10/Clock3 ==
  clock : Inport
  "Reset " : Inport  Port=2
  Memory2 : Memory
  NOT1 : Logic  Operator=NOT  IconShape=distinctive  AllPortsSameDT=off  OutDataTypeStr=boolean
  Product1 : Product
  Triggered Subsystem1 : Subsystem  TreatAsAtomicUnit=on
  T : Outport  VectorParamsAs1DForOutWhenUnconnected=off
  wires:
  Memory2/1 -> Triggered Subsystem1/1(In1)
  Product1/1 -> T/1, Memory2/1
  "Reset "/1 -> NOT1/1
  Triggered Subsystem1/1(Out1) -> Product1/1
  NOT1/1 -> Product1/2
  clock/1 -> Triggered Subsystem1/Trigger

== system pattern3x3_training_2023clock/Synapse10/Subsystem ==
  delta_weight : Inport
  before_weight : Inport  Port=2
  Trigger : TriggerPort  VariantControl=(inherit)  PortDimensions=1
  Sum : Sum  Inputs=|++
  weight : Outport
  wires:
  delta_weight/1 -> Sum/1
  Sum/1 -> weight/1
  before_weight/1 -> Sum/2

== system pattern3x3_training_2023clock/Synapse11/Clock1 ==
  clock : Inport
  "Reset " : Inport  Port=2
  Memory2 : Memory
  NOT1 : Logic  Operator=NOT  IconShape=distinctive  AllPortsSameDT=off  OutDataTypeStr=boolean
  Product1 : Product
  Triggered Subsystem1 : Subsystem  TreatAsAtomicUnit=on
  T : Outport  VectorParamsAs1DForOutWhenUnconnected=off
  wires:
  Memory2/1 -> Triggered Subsystem1/1(In1)
  Product1/1 -> T/1, Memory2/1
  "Reset "/1 -> NOT1/1
  Triggered Subsystem1/1(Out1) -> Product1/1
  NOT1/1 -> Product1/2
  clock/1 -> Triggered Subsystem1/Trigger
